simulink model "power_13NodeTestFeeder_4VSC_PV_DEG_symmtrc_loads_"  (R2024b)
settings: Solver=ode15s  StartTime=0.0  StopTime=5  FixedStep=1e-6  MaxStep=1e-4  RelTol=1e-6  AbsTol=1e-8  EnableMultiTasking=on
PreLoadFcn:
  | %power_13NodeTestFeeder_init;
values from neighbouring files (symbols this model uses):
  a = 1.3    [init_para_with_symmtrc_loads.m]
  Cdc = 278e-3    (= 0.278)    [init_para_with_symmtrc_loads.m]
  fg = 60    [a01_scan_VSC_13_feeder.m]    (also in init_para_with_symmtrc_loads.m)
  Gn = 1000    [init_para_with_symmtrc_loads.m]
  H = 8    [init_para_with_symmtrc_loads.m]
  Ipv_n = Isc_n*(Rp+Rs)/Rp    (= 8.21426513558)    [init_para_with_symmtrc_loads.m]
  Isc_n = 8.21    [init_para_with_symmtrc_loads.m]
  k = 1.3806503e-23    [init_para_with_symmtrc_loads.m]    (also in ypm_plot_compare_ana_meas.m = 2)
  Kdroop = Sn/(Rdroop*60)    (= 4166666.66667)    [init_para_with_symmtrc_loads.m]
  KI = 0.0032    [init_para_with_symmtrc_loads.m]
  Ki_C = Rc/tau_C    (= 0.768)    [init_para_with_symmtrc_loads.m]
  Ki_DC = omega_DC^2*Cdc    [init_para_with_symmtrc_loads.m]
  ki_dvpp = kp_dvpp/Ti_dvpp    [init_para_with_symmtrc_loads.m]
  Ki_P = 1/(Ki_pq*tau_P)    [init_para_with_symmtrc_loads.m]
  Ki_PLL = Kp_PLL/tau_PLL    [init_para_with_symmtrc_loads.m]
  Kp_C = Lc/tau_C    (= 0.020372)    [init_para_with_symmtrc_loads.m]
  Kp_DC = 2*xi_DC*omega_DC*Cdc    [init_para_with_symmtrc_loads.m]
  kp_dvpp = -(2*Kdcgain)^-1    [init_para_with_symmtrc_loads.m]
  Kp_P = tau_C/(Ki_pq*tau_P)    [init_para_with_symmtrc_loads.m]
  Kp_PLL = xi_PLL*2*omega_PLL/Vp    [init_para_with_symmtrc_loads.m]
  KV = -0.123    [init_para_with_symmtrc_loads.m]
  kv_Vp = [ 1.021 1.042 1.0174]    [init_para_with_symmtrc_loads.m]
  KVmp = Vmp_n/Voc_n    (= 0.799392097264)    [init_para_with_symmtrc_loads.m]
  Lc = 20.372e-6    (= 2.0372e-05)    [init_para_with_symmtrc_loads.m]
  Lg = Xg /(2*pi*fg)    [init_para_with_symmtrc_loads.m]
  Np = 345    [init_para_with_symmtrc_loads.m]
  Ns = 45    [init_para_with_symmtrc_loads.m]
  Ns_cell = 54    [init_para_with_symmtrc_loads.m]
  p_jump_time = 5    [init_para_with_symmtrc_loads.m]
  p_jump_value = 2*-1e6    (= -2000000)    [init_para_with_symmtrc_loads.m]
  phi_vec = phi_vec_deg/180*pi    [init_para_with_symmtrc_loads.m]
  ppv_nom = 4.9687e+05    (= 496870)    [init_para_with_symmtrc_loads.m]
  q = 1.6021764e-19    [init_para_with_symmtrc_loads.m]
  Rc = 0.768e-3    (= 0.000768)    [init_para_with_symmtrc_loads.m]
  Rg = (U_rms^2 / S_sc) / (sqrt(1 + XoverR^2))    [init_para_with_symmtrc_loads.m]
  Rp = 425.405    [init_para_with_symmtrc_loads.m]
  Rs = 0.221    [init_para_with_symmtrc_loads.m]
  S_base_all = 1    [init_para_with_symmtrc_loads.m]
  Sn = 15e6    (= 15000000)    [init_para_with_symmtrc_loads.m]
  tau_PLL = 2*xi_PLL/omega_PLL    [init_para_with_symmtrc_loads.m]
  Tn = 25    [init_para_with_symmtrc_loads.m]
  Ts = T_ctrl/n_ctrl    [a01_scan_VSC_13_feeder.m]    (also in init_para_with_symmtrc_loads.m = 5e-05)
  U_rms = 4160    [init_para_with_symmtrc_loads.m]
  Vdc = 1200    [init_para_with_symmtrc_loads.m]
  Voc_n = 32.9    [init_para_with_symmtrc_loads.m]
  Vp = sqrt(2)*480/sqrt(3)    [a01_scan_VSC_13_feeder.m]    (also in init_para_with_symmtrc_loads.m = Ug*sqrt(2)/sqrt(3))
undefined symbols (not defined in the file or in its folder): j, Newton, para_grid, para_PVgeno, Raphson
libraries: spsabctoAlphaBetaZeroLib x141, spsPower3phInstantaneousLib x70, spsSeriesRLCBranchLib x44, spsThreePhaseVIMeasurementLib x27, slpidlib x24, spsThreePhaseSeriesRLCLoadLib x15, spsControlledVoltageSourceLib x15, spsMeanLib x9, spsCurrentMeasurementLib x8, spsControlledCurrentSourceLib x8, cstblocks x8, spsGroundLib x5
(part 3 of 10)

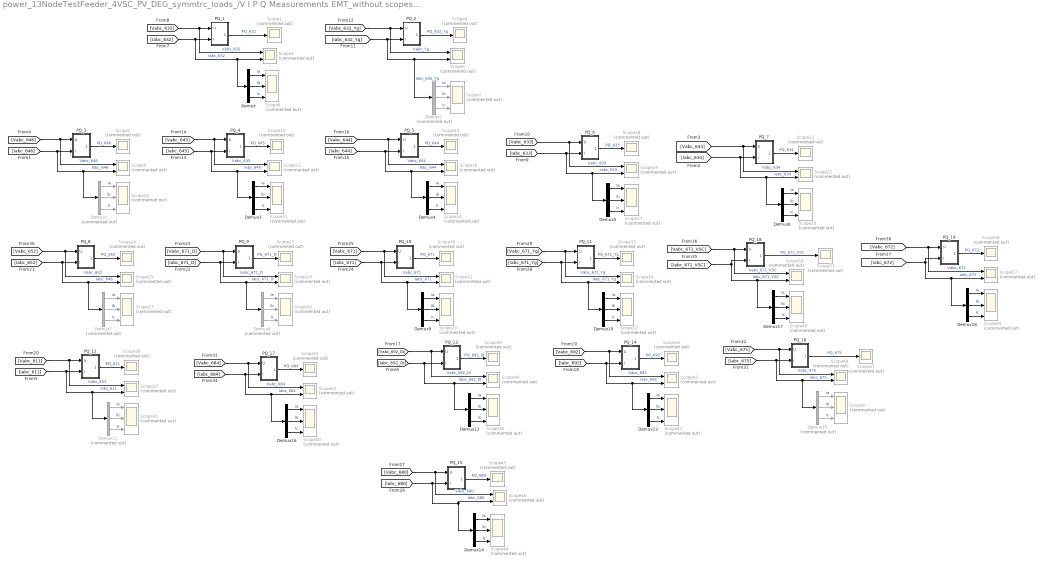
== system power_13NodeTestFeeder_4VSC_PV_DEG_symmtrc_loads_/V I P Q Measurements EMT_without scopes_with_logsout ==
  Demux{,3..6,9..10,12..14,16..18} (13 alike) : Demux  Outputs=3
  Demux{1..2,7..8,11,15} (6 alike) : Demux  Commented=on  Outputs=3
  PQ_1 : Subsystem
  PQ_10 : Subsystem
  PQ_11 : Subsystem
  PQ_12 : Subsystem
  PQ_13 : Subsystem
  PQ_14 : Subsystem
  PQ_15 : Subsystem
  PQ_16 : Subsystem
  PQ_17 : Subsystem
  PQ_18 : Subsystem
  PQ_19 : Subsystem
  PQ_2 : Subsystem
  PQ_3 : Subsystem
  PQ_4 : Subsystem
  PQ_5 : Subsystem
  PQ_6 : Subsystem
  PQ_7 : Subsystem
  PQ_8 : Subsystem
  PQ_9 : Subsystem
  Scope{1..2,4,12,15,18,21,24,27,30,33,36,39,42,45,47,51,53,56} (19 alike) : Scope  Commented=on
  Scope{6..8,10..11,14,17,20,23,26,29,32,35,38,41,44,49..50,55} (19 alike) : Scope  Commented=on  NumInputPorts=3
  Scope{3,5,9,13,16,19,22,25,28,31,34,37,40,43,46,48,52,54,57} (19 alike) : Scope  Commented=on  NumInputPorts=2
  wires:
  [Iabc_632] -> Demux/1, Scope3/2, PQ_1/2(I)  "Iabc_632"
  PQ_1/1(PQ) -> Scope1/1  "PQ_632"
  [Vabc_632] -> Scope3/1, PQ_1/1(U)  "Vabc_632"
  PQ_2/1(PQ) -> Scope4/1  "PQ_632_Yg"
  [Vabc_632_Yg] -> Scope5/1, PQ_2/1(U)  "Vabc_Yg"
  Demux/1 -> Scope6/1  "Ia"
  Demux/2 -> Scope6/2  "Ib"
  Demux/3 -> Scope6/3  "Ic"
  [Iabc_632_Yg] -> Demux1/1, Scope5/2, PQ_2/2(I)  "Iabc_632_Yg"
  Demux1/1 -> Scope7/1  "Ia"
  Demux1/3 -> Scope7/3  "Ic"
  Demux1/2 -> Scope7/2  "Ib"
  Demux2/1 -> Scope10/1  "Ia"
  Demux2/2 -> Scope10/2  "Ib"
  [Iabc_646] -> Scope9/2, Demux2/1, PQ_3/2(I)  "Iabc_646"
  PQ_3/1(PQ) -> Scope2/1  "PQ_646"
  [Vabc_646] -> Scope9/1, PQ_3/1(U)  "Vabc_646"
  Demux2/3 -> Scope10/3  "Ic"
  Demux3/2 -> Scope11/2  "Ib"
  Demux3/1 -> Scope11/1  "Ia"
  Demux3/3 -> Scope11/3  "Ic"
  PQ_4/1(PQ) -> Scope12/1  "PQ_645"
  [Vabc_645] -> Scope13/1, PQ_4/1(U)  "Vabc_645"
  [Iabc_645] -> Scope13/2, Demux3/1, PQ_4/2(I)  "Iabc_645"
  Demux4/2 -> Scope14/2  "Ib"
  Demux4/1 -> Scope14/1  "Ia"
  Demux4/3 -> Scope14/3  "Ic"
  PQ_5/1(PQ) -> Scope15/1  "PQ_644"
  [Vabc_644] -> Scope16/1, PQ_5/1(U)  "Vabc_644"
  [Iabc_644] -> Scope16/2, Demux4/1, PQ_5/2(I)  "Iabc_644"
  Demux5/3 -> Scope17/3  "Ic"
  PQ_6/1(PQ) -> Scope18/1  "PQ_633"
  Demux5/1 -> Scope17/1  "Ia"
  [Vabc_633] -> Scope19/1, PQ_6/1(U)  "Vabc_633"
  Demux5/2 -> Scope17/2  "Ib"
  [Iabc_633] -> Scope19/2, Demux5/1, PQ_6/2(I)  "Iabc_633"
  Demux6/2 -> Scope20/2  "Ib"
  PQ_7/1(PQ) -> Scope21/1  "PQ_634"
  Demux6/3 -> Scope20/3  "Ic"
  Demux6/1 -> Scope20/1  "Ia"
  [Iabc_634] -> Scope22/2, Demux6/1, PQ_7/2(I)  "Iabc_634"
  [Vabc_634] -> Scope22/1, PQ_7/1(U)  "Vabc_634"
  Demux7/2 -> Scope23/2  "Ib"
  Demux7/1 -> Scope23/1  "Ia"
  Demux7/3 -> Scope23/3  "Ic"
  PQ_8/1(PQ) -> Scope24/1  "PQ_652"
  [Vabc_652] -> Scope25/1, PQ_8/1(U)  "Vabc_652"
  [Iabc_652] -> Scope25/2, Demux7/1, PQ_8/2(I)  "Iabc_646"
  Demux8/2 -> Scope26/2  "Ib"
  Demux8/1 -> Scope26/1  "Ia"
  Demux8/3 -> Scope26/3  "Ic"
  PQ_9/1(PQ) -> Scope27/1  "PQ_671_D"
  [Vabc_671_D] -> Scope28/1, PQ_9/1(U)  "Vabc_671_D"
  [Iabc_671_D] -> Scope28/2, Demux8/1, PQ_9/2(I)  "Iabc_671_D"
  Demux9/2 -> Scope29/2  "Ib"
  Demux9/1 -> Scope29/1  "Ia"
  Demux9/3 -> Scope29/3  "Ic"
  PQ_10/1(PQ) -> Scope30/1  "PQ_671"
  [Vabc_671] -> Scope31/1, PQ_10/1(U)  "Vabc_671"
  [Iabc_671] -> Scope31/2, Demux9/1, PQ_10/2(I)  "Iabc_671"
  Demux10/2 -> Scope32/2  "Ib"
  Demux10/1 -> Scope32/1  "Ia"
  Demux10/3 -> Scope32/3  "Ic"
  PQ_11/1(PQ) -> Scope33/1  "PQ_671_Yg"
  [Vabc_671_Yg] -> Scope34/1, PQ_11/1(U)  "Vabc_671_Yg"
  [Iabc_671_Yg] -> Scope34/2, Demux10/1, PQ_11/2(I)  "Iabc_671_Yg"
  [Vabc_611] -> Scope37/1, PQ_12/1(U)  "Vabc_652"
  PQ_12/1(PQ) -> Scope36/1  "PQ_611"
  Demux11/3 -> Scope35/3  "Ic"
  Demux11/1 -> Scope35/1  "Ia"
  [Iabc_611] -> Scope37/2, Demux11/1, PQ_12/2(I)  "Iabc_611"
  Demux11/2 -> Scope35/2  "Ib"
  PQ_13/1(PQ) -> Scope39/1  "PQ_692_DI"
  Demux12/3 -> Scope38/3  "Ic"
  [Vabc_692_DI] -> Scope40/1, PQ_13/1(U)  "Vabc_692_DI"
  Demux12/2 -> Scope38/2  "Ib"
  Demux12/1 -> Scope38/1  "Ia"
  [Iabc_692_DI] -> PQ_13/2(I), Scope40/2, Demux12/1  "Iabc_692_DI"
  PQ_14/1(PQ) -> Scope42/1  "PQ_692"
  Demux13/3 -> Scope41/3  "Ic"
  [Vabc_692] -> Scope43/1, PQ_14/1(U)  "Vabc_692"
  Demux13/2 -> Scope41/2  "Ib"
  Demux13/1 -> Scope41/1  "Ia"
  [Iabc_692] -> Scope43/2, Demux13/1, PQ_14/2(I)  "Iabc_692"
  Demux14/1 -> Scope44/1  "Ia"
  [Vabc_680] -> Scope46/1, PQ_15/1(U)  "Vabc_680"
  [Iabc_680] -> Scope46/2, Demux14/1, PQ_15/2(I)  "Iabc_680"
  PQ_15/1(PQ) -> Scope45/1  "PQ_680"
  Demux14/2 -> Scope44/2  "Ib"
  Demux14/3 -> Scope44/3  "Ic"
  Demux15/3 -> Scope8/3  "Ic"
  Demux15/1 -> Scope8/1  "Ia"
  Demux15/2 -> Scope8/2  "Ib"
  [Iabc_675] -> Scope48/2, Demux15/1, PQ_16/2(I)  "Iabc_675"
  [Vabc_675] -> Scope48/1, PQ_16/1(U)  "Vabc_675"
  PQ_16/1(PQ) -> Scope47/1  "PQ_675"
  [Vabc_684] -> Scope52/1, PQ_17/1(U)  "Vabc_684"
  Demux16/1 -> Scope50/1  "Ia"
  Demux16/3 -> Scope50/3  "Ic"
  [Iabc_684] -> Scope52/2, Demux16/1, PQ_17/2(I)  "Iabc_684"
  Demux16/2 -> Scope50/2  "Ib"
  PQ_17/1(PQ) -> Scope51/1  "PQ_684"
  Demux17/1 -> Scope49/1  "Ia"
  PQ_18/1(PQ) -> Scope53/1  "PQ_671_VSC"
  [Vabc_671_VSC] -> Scope54/1, PQ_18/1(U)  "Vabc_671_VSC"
  Demux17/3 -> Scope49/3  "Ic"
  [Iabc_671_VSC] -> PQ_18/2(I), Scope54/2, Demux17/1  "Iabc_671_VSC"
  Demux17/2 -> Scope49/2  "Ib"
  [Vabc_672] -> Scope57/1, PQ_19/1(U)  "Vabc_672"
  Demux18/2 -> Scope55/2  "Ib"
  Demux18/3 -> Scope55/3  "Ic"
  [Iabc_672] -> PQ_19/2(I), Scope57/2, Demux18/1  "Iabc_672"
  PQ_19/1(PQ) -> Scope56/1  "PQ_672"
  Demux18/1 -> Scope55/1  "Ia"

== system power_13NodeTestFeeder_4VSC_PV_DEG_symmtrc_loads_/V I P Q PV_GENO_VSC Measurements ==
  Demux{7..9,12} (4 alike) : Demux  Outputs=3
  PQ_1 : Subsystem
  PQ_2 : Subsystem
  PQ_3 : Subsystem
  PQ_4 : Subsystem
  Scope{1,4,10,13} (4 alike) : Scope  NumInputPorts=3
  Scope{2,5,7,11} (4 alike) : Scope
  Scope{3,6,9,12} (4 alike) : Scope  NumInputPorts=2
  wires:
  PQ_3/1(PQ) -> Scope11/1  "PQ_at_672"
  Demux8/2 -> Scope13/2  "Ib"
  [Vabc_PVG_at_672] -> Scope12/1, PQ_3/1(U)  "Vabc_at_672"
  Demux9/1 -> Scope10/1  "Ia"
  PQ_1/1(PQ) -> Scope5/1  "PQ_at_680"
  [Iabc_PVG_at_675] -> PQ_2/2(I), Scope9/2, Demux8/1  "Iabc_at_675"
  [Iabc_PVG_at_672] -> PQ_3/2(I), Scope12/2, Demux9/1  "Iabc_at_672"
  Demux8/3 -> Scope13/3  "Ic"
  PQ_2/1(PQ) -> Scope7/1  "PQ_at_675"
  Demux9/3 -> Scope10/3  "Ic"
  Demux7/2 -> Scope4/2  "Ib"
  Demux8/1 -> Scope13/1  "Ia"
  [Iabc_PVG_at_680] -> PQ_1/2(I), Scope6/2, Demux7/1  "Iabc_at_680"
  [Vabc_PVG_at_675] -> Scope9/1, PQ_2/1(U)  "Vabc_at_675"
  [Iabc_PVG_at_634] -> Scope3/2, Demux12/1, PQ_4/2(I)  "Iabc_at_634"
  Demux7/1 -> Scope4/1  "Ia"
  Demux9/2 -> Scope10/2  "Ib"
  PQ_4/1(PQ) -> Scope2/1  "PQ_at_634"
  [Vabc_PVG_at_680] -> Scope6/1, PQ_1/1(U)  "Vabc_at_680"
  [Vabc_PVG_at_634] -> Scope3/1, PQ_4/1(U)  "Vabc_at_634"
  Demux7/3 -> Scope4/3  "Ic"
  Demux12/1 -> Scope1/1  "Ia"
  Demux12/3 -> Scope1/3  "Ic"
  Demux12/2 -> Scope1/2  "Ib"

== system power_13NodeTestFeeder_4VSC_PV_DEG_symmtrc_loads_/Dyn_Equivalent of Extended Grid 4.160 kV/u-controlled Voltage Source ==
  u : Inport
  Controlled Voltage Source : spsControlledVoltageSourceLib/Controlled Voltage Source  Initialize=on  Source_Type=AC  Amplitude=kv_Vp(1) * U_rms / sqrt(3) * sqrt(2) * sin(phi_vec(3))  Phase=phi_vec(3)  Frequency=fg  Measurements=Voltage
  Controlled Voltage Source1 : spsControlledVoltageSourceLib/Controlled Voltage Source  Initialize=on  Source_Type=AC  Amplitude="kv_Vp(2) * U_rms / sqrt(3) * sqrt(2)  * sin(phi_vec(2))"  Phase=phi_vec(2)  Frequency=fg  Measurements=None
  Controlled Voltage Source2 : spsControlledVoltageSourceLib/Controlled Voltage Source  Initialize=on  Source_Type=AC  Amplitude="kv_Vp(1) * U_rms / sqrt(3) * sqrt(2)  * sin(phi_vec(1))"  Phase=phi_vec(1)  Frequency=fg  Measurements=None
  Demux : Demux  Outputs=3
  Ground : spsGroundLib/Ground  LConnTagsString=a
  Series RLC Branch : spsSeriesRLCBranchLib/Series RLC Branch  LConnTagsString=__new0  RConnTagsString=__new0  BranchType=R  Resistance=1e3  Inductance=1e-3  SetiL0=off  InitialCurrent=0  Capacitance=1e-6  Setx0=off  InitialVoltage=0  Measurements=None
  L1 : PMIOPort  Side=Right
  L2 : PMIOPort  Port=2  Side=Right
  L3 : PMIOPort  Port=3  Side=Right
  wires:
  u/1 -> Demux/1
  Demux/3 -> Controlled Voltage Source/1
  Demux/2 -> Controlled Voltage Source1/1
  Demux/1 -> Controlled Voltage Source2/1
  connections:
  Controlled Voltage Source/LConn1 -- Series RLC Branch/LConn1 -- Controlled Voltage Source1/LConn1 -- Controlled Voltage Source2/LConn1
  Controlled Voltage Source2/RConn1 -- L1/RConn1
  Controlled Voltage Source1/RConn1 -- L2/RConn1
  Controlled Voltage Source/RConn1 -- L3/RConn1
  Ground/LConn1 -- Series RLC Branch/RConn1

== system power_13NodeTestFeeder_4VSC_PV_DEG_symmtrc_loads_/Measurements DVPP/PQ_1 ==
  U : Inport
  I : Inport  Port=2
  Complex to Magnitude-Angle1 : ComplexToMagnitudeAngle
  Complex to Magnitude-Angle2 : ComplexToMagnitudeAngle
  Complex to Real-Imag : ComplexToRealImag
  Demux : Demux  Outputs=3
  Demux1 : Demux  Outputs=3
  Gain : Gain  Gain=1/S_base_all
  Gain1 : Gain  Gain=j
  Mux : Mux  Inputs=2
  "Power (3ph, Instantaneous)1" : spsPower3phInstantaneousLib/Power (3ph, Instantaneous)
  Real-Imag to Complex : RealImagToComplex
  Real-Imag to Complex1 : RealImagToComplex
  Sum : Sum  Inputs=|++
  Terminator{1,3,5..8} (6 alike) : Terminator
  Transfer Fcn{1..4} (4 alike) : TransferFcn  Denominator=[1e-3 1]
  abc to Alpha-Beta-Zero : spsabctoAlphaBetaZeroLib/abc to Alpha-Beta-Zero
  abc to Alpha-Beta-Zero1 : spsabctoAlphaBetaZeroLib/abc to Alpha-Beta-Zero
  PQ : Outport
  wires:
  I/1 -> abc to Alpha-Beta-Zero1/1, "Power (3ph, Instantaneous)1"/2
  Gain1/1 -> Sum/2
  Complex to Real-Imag/1 -> Mux/1
  Mux/1 -> PQ/1
  "Power (3ph, Instantaneous)1"/2 -> Transfer Fcn2/1
  "Power (3ph, Instantaneous)1"/1 -> Transfer Fcn1/1
  Sum/1 -> Gain/1
  Gain/1 -> Complex to Real-Imag/1
  U/1 -> abc to Alpha-Beta-Zero/1, "Power (3ph, Instantaneous)1"/1
  abc to Alpha-Beta-Zero/1 -> Demux/1
  Demux/1 -> Real-Imag to Complex/1
  Demux/2 -> Real-Imag to Complex/2
  Real-Imag to Complex/1 -> Complex to Magnitude-Angle2/1
  Complex to Magnitude-Angle2/1 -> Transfer Fcn3/1
  Complex to Magnitude-Angle2/2 -> Terminator3/1
  Complex to Magnitude-Angle1/1 -> Transfer Fcn4/1
  Real-Imag to Complex1/1 -> Complex to Magnitude-Angle1/1
  Demux1/2 -> Real-Imag to Complex1/2
  Demux1/1 -> Real-Imag to Complex1/1
  abc to Alpha-Beta-Zero1/1 -> Demux1/1
  Transfer Fcn1/1 -> Sum/1  "p"
  Transfer Fcn2/1 -> Gain1/1  "p"
  Transfer Fcn3/1 -> Terminator6/1  "u_betrag"
  Transfer Fcn4/1 -> Terminator5/1  "i_betrag"
  Demux1/3 -> Terminator7/1
  Demux/3 -> Terminator8/1
  Complex to Magnitude-Angle1/2 -> Terminator1/1
  Complex to Real-Imag/2 -> Mux/2

== system power_13NodeTestFeeder_4VSC_PV_DEG_symmtrc_loads_/Measurements DVPP/PQ_15 ==
  U : Inport
  I : Inport  Port=2
  Complex to Magnitude-Angle1 : ComplexToMagnitudeAngle
  Complex to Magnitude-Angle2 : ComplexToMagnitudeAngle
  Complex to Real-Imag : ComplexToRealImag
  Demux : Demux  Outputs=3
  Demux1 : Demux  Outputs=3
  Gain : Gain  Gain=1/S_base_all
  Gain1 : Gain  Gain=j
  Mux : Mux  Inputs=2
  "Power (3ph, Instantaneous)1" : spsPower3phInstantaneousLib/Power (3ph, Instantaneous)
  Real-Imag to Complex : RealImagToComplex
  Real-Imag to Complex1 : RealImagToComplex
  Sum : Sum  Inputs=|++
  Terminator{1,3,5..8} (6 alike) : Terminator
  Transfer Fcn{1..4} (4 alike) : TransferFcn  Denominator=[1e-3 1]
  abc to Alpha-Beta-Zero : spsabctoAlphaBetaZeroLib/abc to Alpha-Beta-Zero
  abc to Alpha-Beta-Zero1 : spsabctoAlphaBetaZeroLib/abc to Alpha-Beta-Zero
  PQ : Outport
  wires:
  I/1 -> abc to Alpha-Beta-Zero1/1, "Power (3ph, Instantaneous)1"/2
  Gain1/1 -> Sum/2
  Complex to Real-Imag/1 -> Mux/1
  Complex to Real-Imag/2 -> Mux/2
  Mux/1 -> PQ/1
  "Power (3ph, Instantaneous)1"/2 -> Transfer Fcn2/1
  "Power (3ph, Instantaneous)1"/1 -> Transfer Fcn1/1
  Sum/1 -> Gain/1
  Gain/1 -> Complex to Real-Imag/1
  U/1 -> abc to Alpha-Beta-Zero/1, "Power (3ph, Instantaneous)1"/1
  abc to Alpha-Beta-Zero/1 -> Demux/1
  Demux/1 -> Real-Imag to Complex/1
  Demux/2 -> Real-Imag to Complex/2
  Real-Imag to Complex/1 -> Complex to Magnitude-Angle2/1
  Complex to Magnitude-Angle2/1 -> Transfer Fcn3/1
  Complex to Magnitude-Angle2/2 -> Terminator3/1
  Complex to Magnitude-Angle1/1 -> Transfer Fcn4/1
  Real-Imag to Complex1/1 -> Complex to Magnitude-Angle1/1
  Demux1/2 -> Real-Imag to Complex1/2
  Demux1/1 -> Real-Imag to Complex1/1
  abc to Alpha-Beta-Zero1/1 -> Demux1/1
  Transfer Fcn1/1 -> Sum/1  "p"
  Transfer Fcn2/1 -> Gain1/1  "p"
  Transfer Fcn3/1 -> Terminator6/1  "u_betrag"
  Transfer Fcn4/1 -> Terminator5/1  "i_betrag"
  Demux1/3 -> Terminator7/1
  Demux/3 -> Terminator8/1
  Complex to Magnitude-Angle1/2 -> Terminator1/1

== system power_13NodeTestFeeder_4VSC_PV_DEG_symmtrc_loads_/Measurements DVPP/PQ_16 ==
  U : Inport
  I : Inport  Port=2
  Complex to Magnitude-Angle1 : ComplexToMagnitudeAngle
  Complex to Magnitude-Angle2 : ComplexToMagnitudeAngle
  Complex to Real-Imag : ComplexToRealImag
  Demux : Demux  Outputs=3
  Demux1 : Demux  Outputs=3
  Gain : Gain  Gain=1/S_base_all
  Gain1 : Gain  Gain=j
  Mux : Mux  Inputs=2
  "Power (3ph, Instantaneous)1" : spsPower3phInstantaneousLib/Power (3ph, Instantaneous)
  Real-Imag to Complex : RealImagToComplex
  Real-Imag to Complex1 : RealImagToComplex
  Sum : Sum  Inputs=|++
  Terminator{1,3,5..8} (6 alike) : Terminator
  Transfer Fcn{1..4} (4 alike) : TransferFcn  Denominator=[1e-3 1]
  abc to Alpha-Beta-Zero : spsabctoAlphaBetaZeroLib/abc to Alpha-Beta-Zero
  abc to Alpha-Beta-Zero1 : spsabctoAlphaBetaZeroLib/abc to Alpha-Beta-Zero
  PQ : Outport
  wires:
  I/1 -> abc to Alpha-Beta-Zero1/1, "Power (3ph, Instantaneous)1"/2
  Gain1/1 -> Sum/2
  Complex to Real-Imag/1 -> Mux/1
  Complex to Real-Imag/2 -> Mux/2
  Mux/1 -> PQ/1
  "Power (3ph, Instantaneous)1"/2 -> Transfer Fcn2/1
  "Power (3ph, Instantaneous)1"/1 -> Transfer Fcn1/1
  Sum/1 -> Gain/1
  Gain/1 -> Complex to Real-Imag/1
  U/1 -> abc to Alpha-Beta-Zero/1, "Power (3ph, Instantaneous)1"/1
  abc to Alpha-Beta-Zero/1 -> Demux/1
  Demux/1 -> Real-Imag to Complex/1
  Demux/2 -> Real-Imag to Complex/2
  Real-Imag to Complex/1 -> Complex to Magnitude-Angle2/1
  Complex to Magnitude-Angle2/1 -> Transfer Fcn3/1
  Complex to Magnitude-Angle2/2 -> Terminator3/1
  Complex to Magnitude-Angle1/1 -> Transfer Fcn4/1
  Real-Imag to Complex1/1 -> Complex to Magnitude-Angle1/1
  Demux1/2 -> Real-Imag to Complex1/2
  Demux1/1 -> Real-Imag to Complex1/1
  abc to Alpha-Beta-Zero1/1 -> Demux1/1
  Transfer Fcn1/1 -> Sum/1  "p"
  Transfer Fcn2/1 -> Gain1/1  "p"
  Transfer Fcn3/1 -> Terminator6/1  "u_betrag"
  Transfer Fcn4/1 -> Terminator5/1  "i_betrag"
  Demux1/3 -> Terminator7/1
  Demux/3 -> Terminator8/1
  Complex to Magnitude-Angle1/2 -> Terminator1/1

== system power_13NodeTestFeeder_4VSC_PV_DEG_symmtrc_loads_/Measurements DVPP/PQ_19 ==
  U : Inport
  I : Inport  Port=2
  Complex to Magnitude-Angle1 : ComplexToMagnitudeAngle
  Complex to Magnitude-Angle2 : ComplexToMagnitudeAngle
  Complex to Real-Imag : ComplexToRealImag
  Demux : Demux  Outputs=3
  Demux1 : Demux  Outputs=3
  Gain : Gain  Gain=1/S_base_all
  Gain1 : Gain  Gain=j
  Mux : Mux  Inputs=2
  "Power (3ph, Instantaneous)1" : spsPower3phInstantaneousLib/Power (3ph, Instantaneous)
  Real-Imag to Complex : RealImagToComplex
  Real-Imag to Complex1 : RealImagToComplex
  Sum : Sum  Inputs=|++
  Terminator{1,3,5..8} (6 alike) : Terminator
  Transfer Fcn{1..4} (4 alike) : TransferFcn  Denominator=[1e-3 1]
  abc to Alpha-Beta-Zero : spsabctoAlphaBetaZeroLib/abc to Alpha-Beta-Zero
  abc to Alpha-Beta-Zero1 : spsabctoAlphaBetaZeroLib/abc to Alpha-Beta-Zero
  PQ : Outport
  wires:
  I/1 -> abc to Alpha-Beta-Zero1/1, "Power (3ph, Instantaneous)1"/2
  Gain1/1 -> Sum/2
  Complex to Real-Imag/1 -> Mux/1
  Complex to Real-Imag/2 -> Mux/2
  Mux/1 -> PQ/1
  "Power (3ph, Instantaneous)1"/2 -> Transfer Fcn2/1
  "Power (3ph, Instantaneous)1"/1 -> Transfer Fcn1/1
  Sum/1 -> Gain/1
  Gain/1 -> Complex to Real-Imag/1
  U/1 -> abc to Alpha-Beta-Zero/1, "Power (3ph, Instantaneous)1"/1
  abc to Alpha-Beta-Zero/1 -> Demux/1
  Demux/1 -> Real-Imag to Complex/1
  Demux/2 -> Real-Imag to Complex/2
  Real-Imag to Complex/1 -> Complex to Magnitude-Angle2/1
  Complex to Magnitude-Angle2/1 -> Transfer Fcn3/1
  Complex to Magnitude-Angle2/2 -> Terminator3/1
  Complex to Magnitude-Angle1/1 -> Transfer Fcn4/1
  Real-Imag to Complex1/1 -> Complex to Magnitude-Angle1/1
  Demux1/2 -> Real-Imag to Complex1/2
  Demux1/1 -> Real-Imag to Complex1/1
  abc to Alpha-Beta-Zero1/1 -> Demux1/1
  Transfer Fcn1/1 -> Sum/1  "p"
  Transfer Fcn2/1 -> Gain1/1  "p"
  Transfer Fcn3/1 -> Terminator6/1  "u_betrag"
  Transfer Fcn4/1 -> Terminator5/1  "i_betrag"
  Demux1/3 -> Terminator7/1
  Demux/3 -> Terminator8/1
  Complex to Magnitude-Angle1/2 -> Terminator1/1

== system power_13NodeTestFeeder_4VSC_PV_DEG_symmtrc_loads_/Measurements DVPP/PQ_7 ==
  U : Inport
  I : Inport  Port=2
  Complex to Magnitude-Angle1 : ComplexToMagnitudeAngle
  Complex to Magnitude-Angle2 : ComplexToMagnitudeAngle
  Complex to Real-Imag : ComplexToRealImag
  Demux : Demux  Outputs=3
  Demux1 : Demux  Outputs=3
  Gain : Gain  Gain=1/S_base_all
  Gain1 : Gain  Gain=j
  Mux : Mux  Inputs=2
  "Power (3ph, Instantaneous)1" : spsPower3phInstantaneousLib/Power (3ph, Instantaneous)
  Real-Imag to Complex : RealImagToComplex
  Real-Imag to Complex1 : RealImagToComplex
  Sum : Sum  Inputs=|++
  Terminator{1,3,5..8} (6 alike) : Terminator
  Transfer Fcn{1..4} (4 alike) : TransferFcn  Denominator=[1e-3 1]
  abc to Alpha-Beta-Zero : spsabctoAlphaBetaZeroLib/abc to Alpha-Beta-Zero
  abc to Alpha-Beta-Zero1 : spsabctoAlphaBetaZeroLib/abc to Alpha-Beta-Zero
  PQ : Outport
  wires:
  I/1 -> abc to Alpha-Beta-Zero1/1, "Power (3ph, Instantaneous)1"/2
  Gain1/1 -> Sum/2
  Complex to Real-Imag/1 -> Mux/1
  Complex to Real-Imag/2 -> Mux/2
  Mux/1 -> PQ/1
  "Power (3ph, Instantaneous)1"/2 -> Transfer Fcn2/1
  "Power (3ph, Instantaneous)1"/1 -> Transfer Fcn1/1
  Sum/1 -> Gain/1
  Gain/1 -> Complex to Real-Imag/1
  U/1 -> abc to Alpha-Beta-Zero/1, "Power (3ph, Instantaneous)1"/1
  abc to Alpha-Beta-Zero/1 -> Demux/1
  Demux/1 -> Real-Imag to Complex/1
  Demux/2 -> Real-Imag to Complex/2
  Real-Imag to Complex/1 -> Complex to Magnitude-Angle2/1
  Complex to Magnitude-Angle2/1 -> Transfer Fcn3/1
  Complex to Magnitude-Angle2/2 -> Terminator3/1
  Complex to Magnitude-Angle1/1 -> Transfer Fcn4/1
  Real-Imag to Complex1/1 -> Complex to Magnitude-Angle1/1
  Demux1/2 -> Real-Imag to Complex1/2
  Demux1/1 -> Real-Imag to Complex1/1
  abc to Alpha-Beta-Zero1/1 -> Demux1/1
  Transfer Fcn1/1 -> Sum/1  "p"
  Transfer Fcn2/1 -> Gain1/1  "p"
  Transfer Fcn3/1 -> Terminator6/1  "u_betrag"
  Transfer Fcn4/1 -> Terminator5/1  "i_betrag"
  Demux1/3 -> Terminator7/1
  Demux/3 -> Terminator8/1
  Complex to Magnitude-Angle1/2 -> Terminator1/1

== system power_13NodeTestFeeder_4VSC_PV_DEG_symmtrc_loads_/Measurements DVPP/Subsystem1 ==
  In1 : Inport
  Gain : Gain  Gain=1/3
  Mean value : spsMeanLib/Mean  Freq=fg  Vinit=Vrms0  Ts=Ts
  Product : Product  InputSameDT=on  SaturateOnIntegerOverflow=on  OutDataTypeStr=Inherit: Same as first input
  Saturation to avoid negative sqrt : Saturate  UpperLimit=Inf  LowerLimit=0
  Sqrt : Sqrt  AlgorithmType=Newton-Raphson
  Sum of Elements : Sum  Inputs=+
  Out1 : Outport
  wires:
  Sqrt/1 -> Sum of Elements/1
  Mean value/1 -> Saturation to avoid negative sqrt/1
  Saturation to avoid negative sqrt/1 -> Sqrt/1
  Product/1 -> Mean value/1
  In1/1 -> Product/2, Product/1
  Sum of Elements/1 -> Gain/1
  Gain/1 -> Out1/1

== system power_13NodeTestFeeder_4VSC_PV_DEG_symmtrc_loads_/Measurements DVPP/Subsystem2 ==
  In1 : Inport
  Gain : Gain  Gain=1/3
  Mean value : spsMeanLib/Mean  Freq=fg  Vinit=Vrms0  Ts=Ts
  Product : Product  InputSameDT=on  SaturateOnIntegerOverflow=on  OutDataTypeStr=Inherit: Same as first input
  Saturation to avoid negative sqrt : Saturate  UpperLimit=Inf  LowerLimit=0
  Sqrt : Sqrt  AlgorithmType=Newton-Raphson
  Sum of Elements : Sum  Inputs=+
  Out1 : Outport
  wires:
  Sqrt/1 -> Sum of Elements/1
  Mean value/1 -> Saturation to avoid negative sqrt/1
  Saturation to avoid negative sqrt/1 -> Sqrt/1
  Product/1 -> Mean value/1
  In1/1 -> Product/2, Product/1
  Sum of Elements/1 -> Gain/1
  Gain/1 -> Out1/1

== system power_13NodeTestFeeder_4VSC_PV_DEG_symmtrc_loads_/Measurements DVPP/Subsystem3 ==
  In1 : Inport
  Gain : Gain  Gain=1/3
  Mean value : spsMeanLib/Mean  Freq=fg  Vinit=Vrms0  Ts=Ts
  Product : Product  InputSameDT=on  SaturateOnIntegerOverflow=on  OutDataTypeStr=Inherit: Same as first input
  Saturation to avoid negative sqrt : Saturate  UpperLimit=Inf  LowerLimit=0
  Sqrt : Sqrt  AlgorithmType=Newton-Raphson
  Sum of Elements : Sum  Inputs=+
  Out1 : Outport
  wires:
  Sqrt/1 -> Sum of Elements/1
  Mean value/1 -> Saturation to avoid negative sqrt/1
  Saturation to avoid negative sqrt/1 -> Sqrt/1
  Product/1 -> Mean value/1
  In1/1 -> Product/2, Product/1
  Sum of Elements/1 -> Gain/1
  Gain/1 -> Out1/1

== system power_13NodeTestFeeder_4VSC_PV_DEG_symmtrc_loads_/Measurements DVPP/Subsystem4 ==
  In1 : Inport
  Gain : Gain  Gain=1/3
  Mean value : spsMeanLib/Mean  Freq=fg  Vinit=Vrms0  Ts=Ts
  Product : Product  InputSameDT=on  SaturateOnIntegerOverflow=on  OutDataTypeStr=Inherit: Same as first input
  Saturation to avoid negative sqrt : Saturate  UpperLimit=Inf  LowerLimit=0
  Sqrt : Sqrt  AlgorithmType=Newton-Raphson
  Sum of Elements : Sum  Inputs=+
  Out1 : Outport
  wires:
  Sqrt/1 -> Sum of Elements/1
  Mean value/1 -> Saturation to avoid negative sqrt/1
  Saturation to avoid negative sqrt/1 -> Sqrt/1
  Product/1 -> Mean value/1
  In1/1 -> Product/2, Product/1
  Sum of Elements/1 -> Gain/1
  Gain/1 -> Out1/1

== system power_13NodeTestFeeder_4VSC_PV_DEG_symmtrc_loads_/Measurements DVPP/Subsystem5 ==
  In1 : Inport
  Gain : Gain  Gain=1/3
  Mean value : spsMeanLib/Mean  Freq=fg  Vinit=Vrms0  Ts=Ts
  Product : Product  InputSameDT=on  SaturateOnIntegerOverflow=on  OutDataTypeStr=Inherit: Same as first input
  Saturation to avoid negative sqrt : Saturate  UpperLimit=Inf  LowerLimit=0
  Sqrt : Sqrt  AlgorithmType=Newton-Raphson
  Sum of Elements : Sum  Inputs=+
  Out1 : Outport
  wires:
  Sqrt/1 -> Sum of Elements/1
  Mean value/1 -> Saturation to avoid negative sqrt/1
  Saturation to avoid negative sqrt/1 -> Sqrt/1
  Product/1 -> Mean value/1
  In1/1 -> Product/2, Product/1
  Sum of Elements/1 -> Gain/1
  Gain/1 -> Out1/1

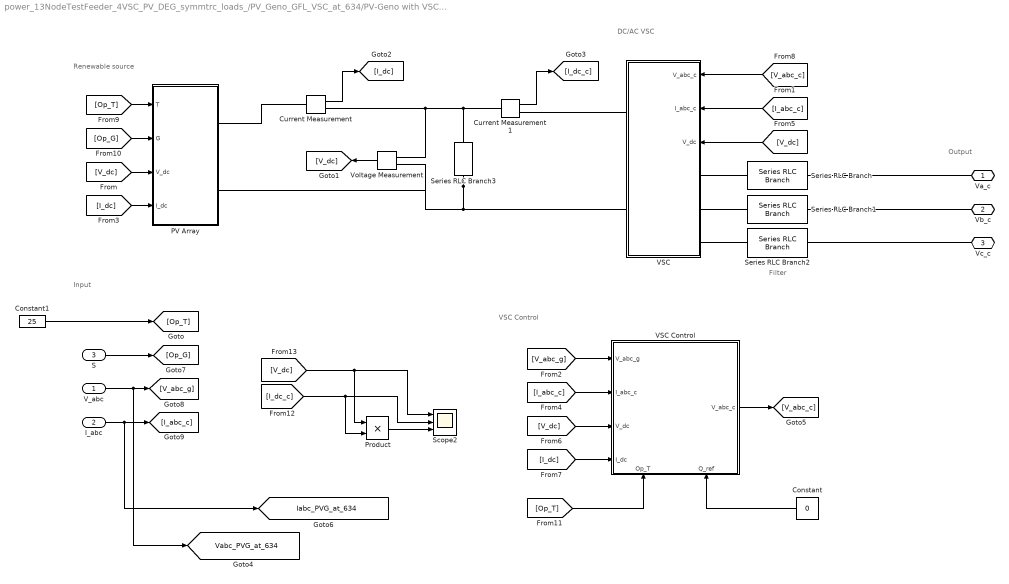
== system power_13NodeTestFeeder_4VSC_PV_DEG_symmtrc_loads_/PV_Geno_GFL_VSC_at_634/PV-Geno with VSC_GFL_at_634      ==
  note: Output
  note: Input
  note: Filter
  note: Renewable source
  note: VSC Control
  note: DC/AC VSC
  V_abc : Inport
  I_abc : Inport  Port=2
  S : Inport  Port=3
  Constant : Constant  Value=0
  Constant1 : Constant  Value=25
  Current Measurement : spsCurrentMeasurementLib/Current Measurement  PhasorSimulation=off  OutputType=Complex  PSBequivalent=0
  Current Measurement1 : spsCurrentMeasurementLib/Current Measurement  PhasorSimulation=off  OutputType=Complex  PSBequivalent=0
  PV Array : Subsystem
  Product : Product
  Scope2 : Scope  NumInputPorts=3
  Series RLC Branch : spsSeriesRLCBranchLib/Series RLC Branch  LConnTagsString=__new0  RConnTagsString=__new0  BranchType=RL  Resistance=Rc  Inductance=Lc  SetiL0=off  InitialCurrent=0  Capacitance=1e-6  Setx0=off  InitialVoltage=0  Measurements=None
  Series RLC Branch1 : spsSeriesRLCBranchLib/Series RLC Branch  LConnTagsString=__new0  RConnTagsString=__new0  BranchType=RL  Resistance=Rc  Inductance=Lc  SetiL0=off  InitialCurrent=0  Capacitance=1e-6  Setx0=off  InitialVoltage=0  Measurements=None
  Series RLC Branch2 : spsSeriesRLCBranchLib/Series RLC Branch  LConnTagsString=__new0  RConnTagsString=__new0  BranchType=RL  Resistance=Rc  Inductance=Lc  SetiL0=off  InitialCurrent=0  Capacitance=1e-6  Setx0=off  InitialVoltage=0  Measurements=None
  Series RLC Branch3 : spsSeriesRLCBranchLib/Series RLC Branch  LConnTagsString=__new0  RConnTagsString=__new0  BranchType=C  Resistance=0.3  Inductance=1e-3  SetiL0=off  InitialCurrent=0  Capacitance=Cdc  Setx0=on  InitialVoltage=Vdc  Measurements=None
  VSC : Subsystem
  VSC Control : Subsystem
      settings: PortSchema="{\"entries\":[{\"content\":{\"sides\":[{\"content\":{\"connectorIds\":[\"In1\",\"In2\",\"In3\",\"In4\"]},\"type\":\"ConnectorPlacement.EquallySpacedRectSide\",\"uuid\":\"1f0c866f-1355-4493-8a8b-fecd52da2e06\"},{\"content\":{\"connectorIds\":[\"Out1\"],\"side\":\"RIGHT\"},\"type\":\"ConnectorPlacement.EquallySpacedRectSide\",\"uuid\":\"e0482316-46fe-491c-835b-46d73fa6817a\"},{\"content\":{\"side\":\"TOP\"},\"type\":\"ConnectorPlacement.EquallySpacedRectSide\",\"uuid\":\"b85aba4d-c629-42a9-b30e-3179992b26cb\"},{\"content\":{\"connectorIds\":[\"In5\",\"In6\"],\"side\":\"BOTTOM\"},\"type\":\"ConnectorPlacement.EquallySpacedRectSide\",\"uuid\":\"2c79aeba-fb98-4b17-8331-d72a75796cf8\"}]},\"type\":\"ConnectorPlacement.EquallySpacedConnector\",\"uuid\":\"5586ce08-6872-4275-b1b0-323c6fc0897a\"}],\"packageUris\":[\"http://schema.mathworks.com/mf0/Connector/R2020b\"],\"version\":\"1.0\"}"
  Voltage Measurement : spsVoltageMeasurementLib/Voltage Measurement  PhasorSimulation=off  OutputType=Complex  PSBequivalent=0
  Va_c : PMIOPort  Side=Left
  Vb_c : PMIOPort  Port=2  Side=Left
  Vc_c : PMIOPort  Port=3  Side=Left
  tag scope: Iabc_PVG_at_634=global, Vabc_PVG_at_634=global
  wires:
  [V_abc_c] -> VSC/1(V_abc_c)
  Constant/1 -> VSC Control/6(Q_ref)
  Current Measurement1/1 -> [I_dc_c]
  [V_dc] -> Scope2/1, Product/1
  [I_dc_c] -> Scope2/2, Product/2
  [I_dc] -> VSC Control/4(I_dc)
  Voltage Measurement/1 -> [V_dc]
  [V_abc_g] -> VSC Control/1(V_abc_g)
  VSC Control/1(V_abc_c) -> [V_abc_c]
  [V_dc] -> PV Array/3(V_dc)
  Current Measurement/1 -> [I_dc]
  Product/1 -> Scope2/3
  [Op_T] -> VSC Control/5(Op_T)
  [V_dc] -> VSC/3(V_dc)
  V_abc/1 -> [Vabc_PVG_at_634], [V_abc_g]
  [Op_T] -> PV Array/1(T)
  [V_dc] -> VSC Control/3(V_dc)
  [Op_G] -> PV Array/2(G)
  [I_abc_c] -> VSC Control/2(I_abc_c)
  [I_abc_c] -> VSC/2(I_abc_c)
  [I_dc] -> PV Array/4(I_dc)
  S/1 -> [Op_G]
  Constant1/1 -> [Op_T]
  I_abc/1 -> [Iabc_PVG_at_634], [I_abc_c]
  connections:
  VSC/LConn2 -- Series RLC Branch1/RConn1
  Series RLC Branch3/RConn1 -- Voltage Measurement/LConn2 -- PV Array/RConn2 -- VSC/RConn2
  Current Measurement1/LConn1 -- Series RLC Branch3/LConn1 -- Current Measurement/RConn1 -- Voltage Measurement/LConn1
  PV Array/RConn1 -- Current Measurement/LConn1
  VSC/LConn1 -- Series RLC Branch/RConn1
  VSC/LConn3 -- Series RLC Branch2/RConn1
  Va_c/RConn1 -- Series RLC Branch/LConn1
  VSC/RConn1 -- Current Measurement1/RConn1
  Vc_c/RConn1 -- Series RLC Branch2/LConn1
  Vb_c/RConn1 -- Series RLC Branch1/LConn1

== system power_13NodeTestFeeder_4VSC_PV_DEG_symmtrc_loads_/PV_Geno_GFL_VSC_at_634/S Signalgenerator_at_1 ==
  Constant : Constant  Value=para_PVgeno.S_ini1
  Product : Product  Commented=on
  Signal Generator : SignalGenerator  Commented=on  Amplitude=50  Frequency=0.25
  Step : Step  Commented=on  Time=para_PVgeno.t_step  After=para_PVgeno.S_step  SampleTime=0
  Step1 : Step  Commented=on  Time=para_PVgeno.t_step11  After=para_PVgeno.S_step11  SampleTime=0
  Step2 : Step  Time=para_PVgeno.t_step12  After=para_PVgeno.S_step12  SampleTime=0
  Sum : Sum  Inputs=|++++
  S : Outport
  wires:
  Sum/1 -> S/1
  Constant/1 -> Sum/1
  Step2/1 -> Sum/3
  Step1/1 -> Product/1
  Signal Generator/1 -> Product/2
  Product/1 -> Sum/2
  Step/1 -> Sum/4

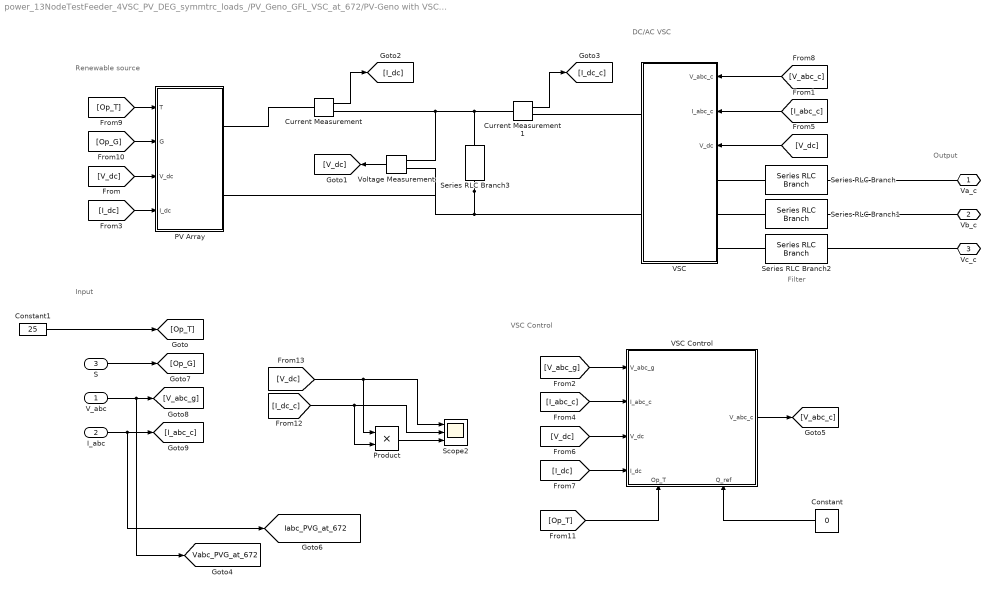
== system power_13NodeTestFeeder_4VSC_PV_DEG_symmtrc_loads_/PV_Geno_GFL_VSC_at_672/PV-Geno with VSC_GFL_at_672 ==
  note: Output
  note: Input
  note: Filter
  note: Renewable source
  note: VSC Control
  note: DC/AC VSC
  V_abc : Inport
  I_abc : Inport  Port=2
  S : Inport  Port=3
  Constant : Constant  Value=0
  Constant1 : Constant  Value=25
  Current Measurement : spsCurrentMeasurementLib/Current Measurement  PhasorSimulation=off  OutputType=Complex  PSBequivalent=0
  Current Measurement1 : spsCurrentMeasurementLib/Current Measurement  PhasorSimulation=off  OutputType=Complex  PSBequivalent=0
  PV Array : Subsystem
  Product : Product
  Scope2 : Scope  NumInputPorts=3
  Series RLC Branch : spsSeriesRLCBranchLib/Series RLC Branch  LConnTagsString=__new0  RConnTagsString=__new0  BranchType=RL  Resistance=Rc  Inductance=Lc  SetiL0=off  InitialCurrent=0  Capacitance=1e-6  Setx0=off  InitialVoltage=0  Measurements=None
  Series RLC Branch1 : spsSeriesRLCBranchLib/Series RLC Branch  LConnTagsString=__new0  RConnTagsString=__new0  BranchType=RL  Resistance=Rc  Inductance=Lc  SetiL0=off  InitialCurrent=0  Capacitance=1e-6  Setx0=off  InitialVoltage=0  Measurements=None
  Series RLC Branch2 : spsSeriesRLCBranchLib/Series RLC Branch  LConnTagsString=__new0  RConnTagsString=__new0  BranchType=RL  Resistance=Rc  Inductance=Lc  SetiL0=off  InitialCurrent=0  Capacitance=1e-6  Setx0=off  InitialVoltage=0  Measurements=None
  Series RLC Branch3 : spsSeriesRLCBranchLib/Series RLC Branch  LConnTagsString=__new0  RConnTagsString=__new0  BranchType=C  Resistance=0.3  Inductance=1e-3  SetiL0=off  InitialCurrent=0  Capacitance=Cdc  Setx0=on  InitialVoltage=Vdc  Measurements=None
  VSC : Subsystem
  VSC Control : Subsystem
      settings: PortSchema="{\"entries\":[{\"content\":{\"sides\":[{\"content\":{\"connectorIds\":[\"In1\",\"In2\",\"In3\",\"In4\"]},\"type\":\"ConnectorPlacement.EquallySpacedRectSide\",\"uuid\":\"1f0c866f-1355-4493-8a8b-fecd52da2e06\"},{\"content\":{\"connectorIds\":[\"Out1\"],\"side\":\"RIGHT\"},\"type\":\"ConnectorPlacement.EquallySpacedRectSide\",\"uuid\":\"e0482316-46fe-491c-835b-46d73fa6817a\"},{\"content\":{\"side\":\"TOP\"},\"type\":\"ConnectorPlacement.EquallySpacedRectSide\",\"uuid\":\"b85aba4d-c629-42a9-b30e-3179992b26cb\"},{\"content\":{\"connectorIds\":[\"In5\",\"In6\"],\"side\":\"BOTTOM\"},\"type\":\"ConnectorPlacement.EquallySpacedRectSide\",\"uuid\":\"2c79aeba-fb98-4b17-8331-d72a75796cf8\"}]},\"type\":\"ConnectorPlacement.EquallySpacedConnector\",\"uuid\":\"5586ce08-6872-4275-b1b0-323c6fc0897a\"}],\"packageUris\":[\"http://schema.mathworks.com/mf0/Connector/R2020b\"],\"version\":\"1.0\"}"
  Voltage Measurement : spsVoltageMeasurementLib/Voltage Measurement  PhasorSimulation=off  OutputType=Complex  PSBequivalent=0
  Va_c : PMIOPort  Side=Left
  Vb_c : PMIOPort  Port=2  Side=Left
  Vc_c : PMIOPort  Port=3  Side=Left
  tag scope: Iabc_PVG_at_672=global, Vabc_PVG_at_672=global
  wires:
  [V_abc_c] -> VSC/1(V_abc_c)
  Constant/1 -> VSC Control/6(Q_ref)
  Current Measurement1/1 -> [I_dc_c]
  [V_dc] -> Scope2/1, Product/1
  [I_dc_c] -> Scope2/2, Product/2
  [I_dc] -> VSC Control/4(I_dc)
  Voltage Measurement/1 -> [V_dc]
  [V_abc_g] -> VSC Control/1(V_abc_g)
  VSC Control/1(V_abc_c) -> [V_abc_c]
  [V_dc] -> PV Array/3(V_dc)
  Current Measurement/1 -> [I_dc]
  Product/1 -> Scope2/3
  [Op_T] -> VSC Control/5(Op_T)
  [V_dc] -> VSC/3(V_dc)
  V_abc/1 -> [Vabc_PVG_at_672], [V_abc_g]
  [Op_T] -> PV Array/1(T)
  [V_dc] -> VSC Control/3(V_dc)
  [Op_G] -> PV Array/2(G)
  [I_abc_c] -> VSC Control/2(I_abc_c)
  [I_abc_c] -> VSC/2(I_abc_c)
  [I_dc] -> PV Array/4(I_dc)
  S/1 -> [Op_G]
  Constant1/1 -> [Op_T]
  I_abc/1 -> [Iabc_PVG_at_672], [I_abc_c]
  connections:
  VSC/LConn2 -- Series RLC Branch1/RConn1
  Series RLC Branch3/RConn1 -- Voltage Measurement/LConn2 -- PV Array/RConn2 -- VSC/RConn2
  Current Measurement1/LConn1 -- Series RLC Branch3/LConn1 -- Current Measurement/RConn1 -- Voltage Measurement/LConn1
  PV Array/RConn1 -- Current Measurement/LConn1
  VSC/LConn1 -- Series RLC Branch/RConn1
  VSC/LConn3 -- Series RLC Branch2/RConn1
  Va_c/RConn1 -- Series RLC Branch/LConn1
  VSC/RConn1 -- Current Measurement1/RConn1
  Vc_c/RConn1 -- Series RLC Branch2/LConn1
  Vb_c/RConn1 -- Series RLC Branch1/LConn1

== system power_13NodeTestFeeder_4VSC_PV_DEG_symmtrc_loads_/PV_Geno_GFL_VSC_at_672/S Signalgenerator_at_672 ==
  Constant : Constant  Value=para_PVgeno.S_ini2
  Product : Product  Commented=on
  Signal Generator : SignalGenerator  Commented=on  Amplitude=0
  Step : Step  Commented=on  Time=para_PVgeno.t_step  After=para_PVgeno.S_step  SampleTime=0
  Step1 : Step  Commented=on  Time=para_PVgeno.t_step21  After=para_PVgeno.S_step21  SampleTime=0
  Step2 : Step  Time=para_PVgeno.t_step22  After=para_PVgeno.S_step22  SampleTime=0
  Sum : Sum  Inputs=|++++
  S : Outport
  wires:
  Product/1 -> Sum/2
  Sum/1 -> S/1
  Constant/1 -> Sum/1
  Signal Generator/1 -> Product/2
  Step2/1 -> Sum/3
  Step1/1 -> Product/1
  Step/1 -> Sum/4

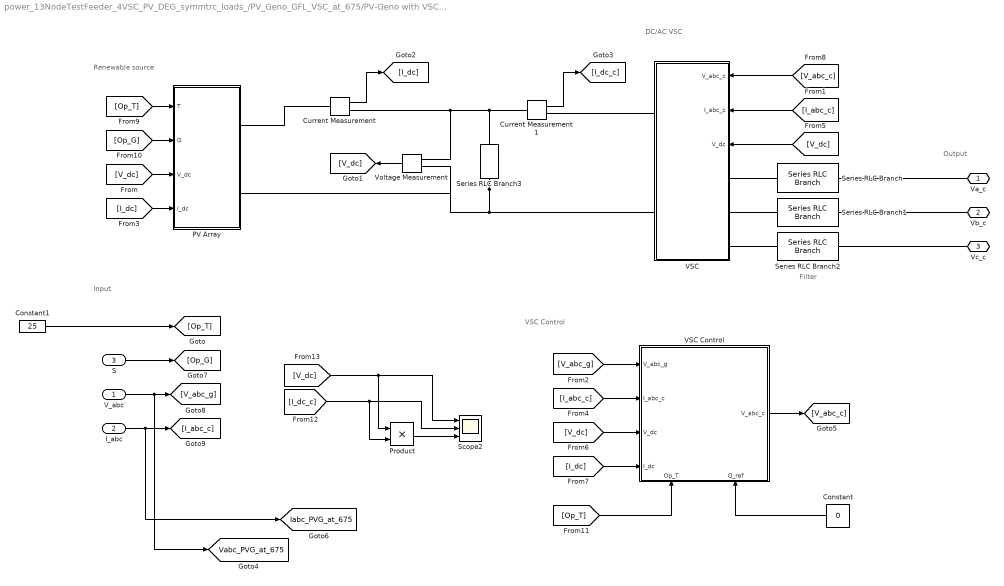
== system power_13NodeTestFeeder_4VSC_PV_DEG_symmtrc_loads_/PV_Geno_GFL_VSC_at_675/PV-Geno with VSC_GFL_at_675 ==
  note: Output
  note: Input
  note: Filter
  note: Renewable source
  note: VSC Control
  note: DC/AC VSC
  V_abc : Inport
  I_abc : Inport  Port=2
  S : Inport  Port=3
  Constant : Constant  Value=0
  Constant1 : Constant  Value=25
  Current Measurement : spsCurrentMeasurementLib/Current Measurement  PhasorSimulation=off  OutputType=Complex  PSBequivalent=0
  Current Measurement1 : spsCurrentMeasurementLib/Current Measurement  PhasorSimulation=off  OutputType=Complex  PSBequivalent=0
  PV Array : Subsystem
  Product : Product
  Scope2 : Scope  NumInputPorts=3
  Series RLC Branch : spsSeriesRLCBranchLib/Series RLC Branch  LConnTagsString=__new0  RConnTagsString=__new0  BranchType=RL  Resistance=Rc  Inductance=Lc  SetiL0=off  InitialCurrent=0  Capacitance=1e-6  Setx0=off  InitialVoltage=0  Measurements=None
  Series RLC Branch1 : spsSeriesRLCBranchLib/Series RLC Branch  LConnTagsString=__new0  RConnTagsString=__new0  BranchType=RL  Resistance=Rc  Inductance=Lc  SetiL0=off  InitialCurrent=0  Capacitance=1e-6  Setx0=off  InitialVoltage=0  Measurements=None
  Series RLC Branch2 : spsSeriesRLCBranchLib/Series RLC Branch  LConnTagsString=__new0  RConnTagsString=__new0  BranchType=RL  Resistance=Rc  Inductance=Lc  SetiL0=off  InitialCurrent=0  Capacitance=1e-6  Setx0=off  InitialVoltage=0  Measurements=None
  Series RLC Branch3 : spsSeriesRLCBranchLib/Series RLC Branch  LConnTagsString=__new0  RConnTagsString=__new0  BranchType=C  Resistance=0.3  Inductance=1e-3  SetiL0=off  InitialCurrent=0  Capacitance=Cdc  Setx0=on  InitialVoltage=Vdc  Measurements=None
  VSC : Subsystem
  VSC Control : Subsystem
      settings: PortSchema="{\"entries\":[{\"content\":{\"sides\":[{\"content\":{\"connectorIds\":[\"In1\",\"In2\",\"In3\",\"In4\"]},\"type\":\"ConnectorPlacement.EquallySpacedRectSide\",\"uuid\":\"1f0c866f-1355-4493-8a8b-fecd52da2e06\"},{\"content\":{\"connectorIds\":[\"Out1\"],\"side\":\"RIGHT\"},\"type\":\"ConnectorPlacement.EquallySpacedRectSide\",\"uuid\":\"e0482316-46fe-491c-835b-46d73fa6817a\"},{\"content\":{\"side\":\"TOP\"},\"type\":\"ConnectorPlacement.EquallySpacedRectSide\",\"uuid\":\"b85aba4d-c629-42a9-b30e-3179992b26cb\"},{\"content\":{\"connectorIds\":[\"In5\",\"In6\"],\"side\":\"BOTTOM\"},\"type\":\"ConnectorPlacement.EquallySpacedRectSide\",\"uuid\":\"2c79aeba-fb98-4b17-8331-d72a75796cf8\"}]},\"type\":\"ConnectorPlacement.EquallySpacedConnector\",\"uuid\":\"5586ce08-6872-4275-b1b0-323c6fc0897a\"}],\"packageUris\":[\"http://schema.mathworks.com/mf0/Connector/R2020b\"],\"version\":\"1.0\"}"
  Voltage Measurement : spsVoltageMeasurementLib/Voltage Measurement  PhasorSimulation=off  OutputType=Complex  PSBequivalent=0
  Va_c : PMIOPort  Side=Left
  Vb_c : PMIOPort  Port=2  Side=Left
  Vc_c : PMIOPort  Port=3  Side=Left
  tag scope: Iabc_PVG_at_675=global, Vabc_PVG_at_675=global
  wires:
  [V_abc_c] -> VSC/1(V_abc_c)
  Constant/1 -> VSC Control/6(Q_ref)
  Current Measurement1/1 -> [I_dc_c]
  [V_dc] -> Scope2/1, Product/1
  [I_dc_c] -> Scope2/2, Product/2
  [I_dc] -> VSC Control/4(I_dc)
  Voltage Measurement/1 -> [V_dc]
  [V_abc_g] -> VSC Control/1(V_abc_g)
  VSC Control/1(V_abc_c) -> [V_abc_c]
  [V_dc] -> PV Array/3(V_dc)
  Current Measurement/1 -> [I_dc]
  Product/1 -> Scope2/3
  [Op_T] -> VSC Control/5(Op_T)
  [V_dc] -> VSC/3(V_dc)
  V_abc/1 -> [Vabc_PVG_at_675], [V_abc_g]
  [Op_T] -> PV Array/1(T)
  [V_dc] -> VSC Control/3(V_dc)
  [Op_G] -> PV Array/2(G)
  [I_abc_c] -> VSC Control/2(I_abc_c)
  [I_abc_c] -> VSC/2(I_abc_c)
  [I_dc] -> PV Array/4(I_dc)
  S/1 -> [Op_G]
  Constant1/1 -> [Op_T]
  I_abc/1 -> [Iabc_PVG_at_675], [I_abc_c]
  connections:
  VSC/LConn2 -- Series RLC Branch1/RConn1
  Series RLC Branch3/RConn1 -- Voltage Measurement/LConn2 -- PV Array/RConn2 -- VSC/RConn2
  Current Measurement1/LConn1 -- Series RLC Branch3/LConn1 -- Current Measurement/RConn1 -- Voltage Measurement/LConn1
  PV Array/RConn1 -- Current Measurement/LConn1
  VSC/LConn1 -- Series RLC Branch/RConn1
  VSC/LConn3 -- Series RLC Branch2/RConn1
  Va_c/RConn1 -- Series RLC Branch/LConn1
  VSC/RConn1 -- Current Measurement1/RConn1
  Vc_c/RConn1 -- Series RLC Branch2/LConn1
  Vb_c/RConn1 -- Series RLC Branch1/LConn1

== system power_13NodeTestFeeder_4VSC_PV_DEG_symmtrc_loads_/PV_Geno_GFL_VSC_at_675/S Signalgenerator_at_675 ==
  Constant : Constant  Value=para_PVgeno.S_ini3
  Product : Product  Commented=on
  Signal Generator : SignalGenerator  Commented=on  Amplitude=0
  Step : Step  Commented=on  Time=para_PVgeno.t_step  After=para_PVgeno.S_step  SampleTime=0
  Step1 : Step  Commented=on  Time=para_PVgeno.t_step31  After=para_PVgeno.S_step31  SampleTime=0
  Step2 : Step  Time=para_PVgeno.t_step32  After=para_PVgeno.S_step32  SampleTime=0
  Sum : Sum  Inputs=|++++
  S : Outport
  wires:
  Product/1 -> Sum/2
  Sum/1 -> S/1
  Constant/1 -> Sum/1
  Signal Generator/1 -> Product/2
  Step2/1 -> Sum/3
  Step1/1 -> Product/1
  Step/1 -> Sum/4

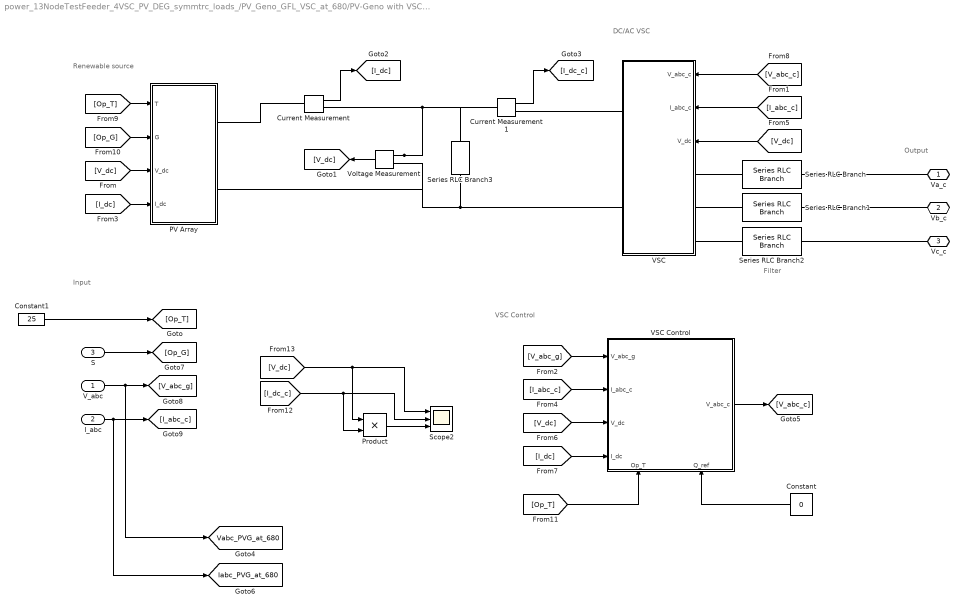
== system power_13NodeTestFeeder_4VSC_PV_DEG_symmtrc_loads_/PV_Geno_GFL_VSC_at_680/PV-Geno with VSC_GFL_at_680 ==
  note: DC/AC VSC
  note: VSC Control
  note: Renewable source
  note: Filter
  note: Input
  note: Output
  V_abc : Inport
  I_abc : Inport  Port=2
  S : Inport  Port=3
  Constant : Constant  Value=0
  Constant1 : Constant  Value=25
  Current Measurement : spsCurrentMeasurementLib/Current Measurement  PhasorSimulation=off  OutputType=Complex  PSBequivalent=0
  Current Measurement1 : spsCurrentMeasurementLib/Current Measurement  PhasorSimulation=off  OutputType=Complex  PSBequivalent=0
  PV Array : Subsystem
  Product : Product
  Scope2 : Scope  NumInputPorts=3
  Series RLC Branch : spsSeriesRLCBranchLib/Series RLC Branch  LConnTagsString=__new0  RConnTagsString=__new0  BranchType=RL  Resistance=Rc  Inductance=Lc  SetiL0=off  InitialCurrent=0  Capacitance=1e-6  Setx0=off  InitialVoltage=0  Measurements=None
  Series RLC Branch1 : spsSeriesRLCBranchLib/Series RLC Branch  LConnTagsString=__new0  RConnTagsString=__new0  BranchType=RL  Resistance=Rc  Inductance=Lc  SetiL0=off  InitialCurrent=0  Capacitance=1e-6  Setx0=off  InitialVoltage=0  Measurements=None
  Series RLC Branch2 : spsSeriesRLCBranchLib/Series RLC Branch  LConnTagsString=__new0  RConnTagsString=__new0  BranchType=RL  Resistance=Rc  Inductance=Lc  SetiL0=off  InitialCurrent=0  Capacitance=1e-6  Setx0=off  InitialVoltage=0  Measurements=None
  Series RLC Branch3 : spsSeriesRLCBranchLib/Series RLC Branch  LConnTagsString=__new0  RConnTagsString=__new0  BranchType=C  Resistance=0.3  Inductance=1e-3  SetiL0=off  InitialCurrent=0  Capacitance=Cdc  Setx0=on  InitialVoltage=Vdc  Measurements=None
  VSC : Subsystem
  VSC Control : Subsystem
      settings: PortSchema="{\"entries\":[{\"content\":{\"sides\":[{\"content\":{\"connectorIds\":[\"In1\",\"In2\",\"In3\",\"In4\"]},\"type\":\"ConnectorPlacement.EquallySpacedRectSide\",\"uuid\":\"1f0c866f-1355-4493-8a8b-fecd52da2e06\"},{\"content\":{\"connectorIds\":[\"Out1\"],\"side\":\"RIGHT\"},\"type\":\"ConnectorPlacement.EquallySpacedRectSide\",\"uuid\":\"e0482316-46fe-491c-835b-46d73fa6817a\"},{\"content\":{\"side\":\"TOP\"},\"type\":\"ConnectorPlacement.EquallySpacedRectSide\",\"uuid\":\"b85aba4d-c629-42a9-b30e-3179992b26cb\"},{\"content\":{\"connectorIds\":[\"In5\",\"In6\"],\"side\":\"BOTTOM\"},\"type\":\"ConnectorPlacement.EquallySpacedRectSide\",\"uuid\":\"2c79aeba-fb98-4b17-8331-d72a75796cf8\"}]},\"type\":\"ConnectorPlacement.EquallySpacedConnector\",\"uuid\":\"5586ce08-6872-4275-b1b0-323c6fc0897a\"}],\"packageUris\":[\"http://schema.mathworks.com/mf0/Connector/R2020b\"],\"version\":\"1.0\"}"
  Voltage Measurement : spsVoltageMeasurementLib/Voltage Measurement  PhasorSimulation=off  OutputType=Complex  PSBequivalent=0
  Va_c : PMIOPort  Side=Left
  Vb_c : PMIOPort  Port=2  Side=Left
  Vc_c : PMIOPort  Port=3  Side=Left
  tag scope: Iabc_PVG_at_680=global, Vabc_PVG_at_680=global
  wires:
  Constant1/1 -> [Op_T]
  S/1 -> [Op_G]
  [I_dc] -> PV Array/4(I_dc)
  [I_abc_c] -> VSC/2(I_abc_c)
  [I_abc_c] -> VSC Control/2(I_abc_c)
  [Op_G] -> PV Array/2(G)
  [V_dc] -> VSC Control/3(V_dc)
  [Op_T] -> PV Array/1(T)
  V_abc/1 -> [Vabc_PVG_at_680], [V_abc_g]
  [V_dc] -> VSC/3(V_dc)
  [Op_T] -> VSC Control/5(Op_T)
  Product/1 -> Scope2/3
  Current Measurement/1 -> [I_dc]
  [V_dc] -> PV Array/3(V_dc)
  VSC Control/1(V_abc_c) -> [V_abc_c]
  [V_abc_g] -> VSC Control/1(V_abc_g)
  Voltage Measurement/1 -> [V_dc]
  [I_dc] -> VSC Control/4(I_dc)
  [I_dc_c] -> Product/2, Scope2/2
  [V_dc] -> Product/1, Scope2/1
  Current Measurement1/1 -> [I_dc_c]
  I_abc/1 -> [Iabc_PVG_at_680], [I_abc_c]
  Constant/1 -> VSC Control/6(Q_ref)
  [V_abc_c] -> VSC/1(V_abc_c)
  connections:
  Vb_c/RConn1 -- Series RLC Branch1/LConn1
  Vc_c/RConn1 -- Series RLC Branch2/LConn1
  VSC/RConn1 -- Current Measurement1/RConn1
  Va_c/RConn1 -- Series RLC Branch/LConn1
  VSC/LConn3 -- Series RLC Branch2/RConn1
  VSC/LConn1 -- Series RLC Branch/RConn1
  PV Array/RConn1 -- Current Measurement/LConn1
  Voltage Measurement/LConn1 -- Current Measurement/RConn1 -- Series RLC Branch3/LConn1 -- Current Measurement1/LConn1
  VSC/RConn2 -- PV Array/RConn2 -- Voltage Measurement/LConn2 -- Series RLC Branch3/RConn1
  VSC/LConn2 -- Series RLC Branch1/RConn1

== system power_13NodeTestFeeder_4VSC_PV_DEG_symmtrc_loads_/PV_Geno_GFL_VSC_at_680/S Signalgenerator_at_680 ==
  Constant : Constant  Value=para_PVgeno.S_ini4
  Product : Product  Commented=on
  Signal Generator : SignalGenerator  Commented=on  Amplitude=0
  Step : Step  Commented=on  Time=para_PVgeno.t_step  After=para_PVgeno.S_step  SampleTime=0
  Step1 : Step  Commented=on  Time=para_PVgeno.t_step41  After=para_PVgeno.S_step41  SampleTime=0
  Step2 : Step  Time=para_PVgeno.t_step42  After=para_PVgeno.S_step42  SampleTime=0
  Sum : Sum  Inputs=|++++
  S : Outport
  wires:
  Product/1 -> Sum/2
  Sum/1 -> S/1
  Constant/1 -> Sum/1
  Signal Generator/1 -> Product/2
  Step2/1 -> Sum/3
  Step1/1 -> Product/1
  Step/1 -> Sum/4

== system power_13NodeTestFeeder_4VSC_PV_DEG_symmtrc_loads_/RMS and Pos // Neg Sequence Calculation /Subsystem ==
  Vabc_634 : Inport
  Iabc_634 : Inport  Port=2
  PLL aligned with positive-sequence : Subsystem
  Phase-sequence separation1 : Subsystem
  Phase-sequence separation2 : Subsystem
  vq+ : Outport
  vd+ : Outport  Port=2
  vq- : Outport  Port=3
  vd- : Outport  Port=4
  iq+ : Outport  Port=5
  id+ : Outport  Port=6
  iq- : Outport  Port=7
  id- : Outport  Port=8
  f_PLL : Outport  Port=9
  wires:
  Phase-sequence separation1/2(d+) -> id+/1  "id+"
  PLL aligned with positive-sequence/2(f) -> f_PLL/1  "f_PLL"
  Phase-sequence separation2/2(d+) -> vd+/1  "vd+"
  Phase-sequence separation2/1(q+) -> vq+/1  "vq+"
  Phase-sequence separation2/4(d-) -> vd-/1  "vd-"
  PLL aligned with positive-sequence/1(theta) -> Phase-sequence separation1/2(Theta), Phase-sequence separation2/2(Theta)  "theta"
  Vabc_634/1 -> PLL aligned with positive-sequence/1(Vabc), Phase-sequence separation2/1(abc)
  Phase-sequence separation1/4(d-) -> id-/1  "id-"
  Phase-sequence separation2/3(q-) -> vq-/1  "vq-"
  Iabc_634/1 -> Phase-sequence separation1/1(abc)
  Phase-sequence separation1/1(q+) -> iq+/1  "iq+"
  Phase-sequence separation1/3(q-) -> iq-/1  "iq-"

== system power_13NodeTestFeeder_4VSC_PV_DEG_symmtrc_loads_/RMS and Pos // Neg Sequence Calculation /Subsystem1 ==
  Vabc_645 : Inport
  Iabc_645 : Inport  Port=2
  PLL aligned with positive-sequence : Subsystem
  Phase-sequence separation1 : Subsystem
  Phase-sequence separation2 : Subsystem
  vq+ : Outport
  vd+ : Outport  Port=2
  vq- : Outport  Port=3
  vd- : Outport  Port=4
  iq+ : Outport  Port=5
  id+ : Outport  Port=6
  iq- : Outport  Port=7
  id- : Outport  Port=8
  f_PLL : Outport  Port=9
  wires:
  Phase-sequence separation1/2(d+) -> id+/1  "id+"
  PLL aligned with positive-sequence/2(f) -> f_PLL/1  "f_PLL"
  Phase-sequence separation2/2(d+) -> vd+/1  "vd+"
  Phase-sequence separation2/1(q+) -> vq+/1  "vq+"
  Phase-sequence separation2/4(d-) -> vd-/1  "vd-"
  PLL aligned with positive-sequence/1(theta) -> Phase-sequence separation1/2(Theta), Phase-sequence separation2/2(Theta)  "theta"
  Vabc_645/1 -> PLL aligned with positive-sequence/1(Vabc), Phase-sequence separation2/1(abc)
  Phase-sequence separation1/4(d-) -> id-/1  "id-"
  Phase-sequence separation2/3(q-) -> vq-/1  "vq-"
  Iabc_645/1 -> Phase-sequence separation1/1(abc)
  Phase-sequence separation1/1(q+) -> iq+/1  "iq+"
  Phase-sequence separation1/3(q-) -> iq-/1  "iq-"
